simulink model "power_mosfet_device"  (R2025b)
settings: Solver=ode23tb  StartTime=0.0  StopTime=simlength  MaxStep=tc  RelTol=1e-3
values from neighbouring files (symbols this model uses):
  freq = 20e3    (= 20000)    [init_model.m]
  m = 0.5    [init_model.m]
  Rgate_turn_off = 1e-3    (= 0.001)    [init_model.m]
  Rgate_turn_on = 1    [init_model.m]
undefined symbols (not defined in the file or in its folder): cp_al, DThs_init, mosfet, Rth_mosfet_HA, Tambient, weigth
libraries: fl_lib x68, nesl_utility x32, simulink x4, advanced_mosfet_lib x2, basic_mosfet_lib x1, ee_lib x1
(part 2 of 2)

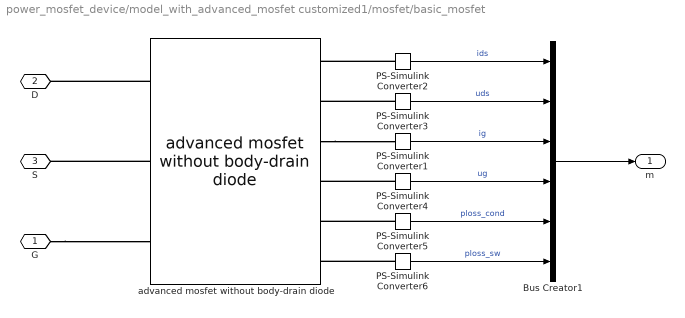
== system power_mosfet_device/model_with_advanced_mosfet customized1/mosfet/basic_mosfet ==
  Bus Creator1 : BusCreator  Inputs=6
  PS-Simulink Converter1 : nesl_utility/PS-Simulink Converter  PhysicalDomain=network_engine_domain  SubClassName=ps_output  LeftPortType=input  RightPortType=output  PseudoPeriodic=off  Frequencies=[]  VectorFormat=1-D array  Unit=A  AffineConversion=off
  PS-Simulink Converter2 : nesl_utility/PS-Simulink Converter  PhysicalDomain=network_engine_domain  SubClassName=ps_output  LeftPortType=input  RightPortType=output  PseudoPeriodic=off  Frequencies=[]  VectorFormat=1-D array  Unit=A  AffineConversion=off
  PS-Simulink Converter3 : nesl_utility/PS-Simulink Converter  PhysicalDomain=network_engine_domain  SubClassName=ps_output  LeftPortType=input  RightPortType=output  PseudoPeriodic=off  Frequencies=[]  VectorFormat=1-D array  Unit=V  AffineConversion=off
  PS-Simulink Converter4 : nesl_utility/PS-Simulink Converter  PhysicalDomain=network_engine_domain  SubClassName=ps_output  LeftPortType=input  RightPortType=output  PseudoPeriodic=off  Frequencies=[]  VectorFormat=1-D array  Unit=V  AffineConversion=off
  PS-Simulink Converter5 : nesl_utility/PS-Simulink Converter  PhysicalDomain=network_engine_domain  SubClassName=ps_output  LeftPortType=input  RightPortType=output  PseudoPeriodic=off  Frequencies=[]  VectorFormat=1-D array  Unit=W  AffineConversion=off
  PS-Simulink Converter6 : nesl_utility/PS-Simulink Converter  PhysicalDomain=network_engine_domain  SubClassName=ps_output  LeftPortType=input  RightPortType=output  PseudoPeriodic=off  Frequencies=[]  VectorFormat=1-D array  Unit=W  AffineConversion=off
  advanced mosfet without body-drain diode : advanced_mosfet_lib/advanced mosfet without body-drain diode  Vth=Vth_m V  g_fs=g_fs_m A/V  Rds_on=Rds_on_m Ohm  Cgs=Cgs_m F  Cgd=Cgd_m F  Cds=Cds_m F  Rg=Rgate_internal_m Ohm  Eon=Eon_m J  Eoff=Eoff_m J  Err=Err_m J  Voff_sw_loss=Voff_sw_loss_m V  Ion_sw_loss=Ion_sw_loss_m A  ids_i_specify=off  ids_i_priority=None  ids_i=0 A  ids_i_nominal_specify=off  ids_i_nominal_value=1  ids_i_nominal_unit=A  ids_ii_specify=off  ids_ii_priority=None  ids_ii=0 A  ids_ii_nominal_specify=off  ids_ii_nominal_value=1  ids_ii_nominal_unit=A  idsi_specify=off  idsi_priority=High  idsi=0 A  idsi_nominal_specify=off  idsi_nominal_value=1  idsi_nominal_unit=A  icgs_specify=off  icgs_priority=None  icgs=0 A  icgs_nominal_specify=off  icgs_nominal_value=1  icgs_nominal_unit=A  icgd_specify=off  icgd_priority=None  icgd=0 A  icgd_nominal_specify=off  icgd_nominal_value=1  icgd_nominal_unit=A  icds_specify=off  icds_priority=None  icds=0 A  icds_nominal_specify=off  icds_nominal_value=1  icds_nominal_unit=A  ugs_specify=off  ugs_priority=None  ugs=0 V  ugs_nominal_specify=off  ugs_nominal_value=1  ugs_nominal_unit=V  uds_specify=off  uds_priority=None  uds=0 V  uds_nominal_specify=off  uds_nominal_value=1  uds_nominal_unit=V  ucgs_specify=off  ucgs_priority=None  ucgs=0 V  ucgs_nominal_specify=off  ucgs_nominal_value=1  ucgs_nominal_unit=V  ucgd_specify=off  ucgd_priority=None  ucgd=0 V  ucgd_nominal_specify=off  ucgd_nominal_value=1  ucgd_nominal_unit=V  udsi_specify=off  udsi_priority=None  udsi=0 V  udsi_nominal_specify=off  udsi_nominal_value=1  udsi_nominal_unit=V  igs_specify=off  igs_priority=High  igs=0 A  igs_nominal_specify=off  igs_nominal_value=1  igs_nominal_unit=A  idsi_active_specify=off  idsi_active_priority=None  idsi_active=0 A  idsi_active_nominal_specify=off  idsi_active_nominal_value=1  idsi_active_nominal_unit=A  idsi_on_specify=off  idsi_on_priority=None  idsi_on=0 A  idsi_on_nominal_specify=off  idsi_on_nominal_value=1  idsi_on_nominal_unit=A
      settings: InternalSimscapePortConfiguration="{\"Bottom\":[],\"Left\":[{\"id\":\"D\",\"label\":\"D\",\"type\":\"foundation.electrical.electrical\"},{\"id\":\"S\",\"label\":\"S\",\"type\":\"foundation.electrical.electrical\"},{\"id\":\"G\",\"label\":\"G\",\"type\":\"foundation.electrical.electrical\"}],\"Right\":[{\"id\":\"idsi_out\",\"label\":\"ids\",\"type\":\"output\"},{\"id\":\"udsi_out\",\"label\":\"uds\",\"type\":\"output\"},{\"id\":\"igs_out\",\"label\":\"igs\",\"type\":\"output\"},{\"id\":\"ugs_out\",\"label\":\"ugs\",\"type\":\"output\"},{\"id\":\"ploss_cond\",\"label\":\"ploss_cond\",\"type\":\"output\"},{\"id\":\"ploss_sw\",\"label\":\"ploss_sw\",\"type\":\"output\"}],\"Top\":[]}"
  G : PMIOPort  Side=Left
  D : PMIOPort  Port=2  Side=Left
  S : PMIOPort  Port=3  Side=Right
  m : Outport
  wires:
  PS-Simulink Converter6/1 -> Bus Creator1/6  "ploss_sw"
  PS-Simulink Converter5/1 -> Bus Creator1/5  "ploss_cond"
  PS-Simulink Converter4/1 -> Bus Creator1/4  "ug"
  PS-Simulink Converter1/1 -> Bus Creator1/3  "ig"
  PS-Simulink Converter3/1 -> Bus Creator1/2  "uds"
  PS-Simulink Converter2/1 -> Bus Creator1/1  "ids"
  Bus Creator1/1 -> m/1
  connections:
  PS-Simulink Converter6/LConn1 -- advanced mosfet without body-drain diode/RConn6
  PS-Simulink Converter5/LConn1 -- advanced mosfet without body-drain diode/RConn5
  advanced mosfet without body-drain diode/RConn3 -- PS-Simulink Converter1/LConn1
  PS-Simulink Converter4/LConn1 -- advanced mosfet without body-drain diode/RConn4
  G/RConn1 -- advanced mosfet without body-drain diode/LConn3
  advanced mosfet without body-drain diode/LConn2 -- S/RConn1
  advanced mosfet without body-drain diode/LConn1 -- D/RConn1
  PS-Simulink Converter2/LConn1 -- advanced mosfet without body-drain diode/RConn1
  PS-Simulink Converter3/LConn1 -- advanced mosfet without body-drain diode/RConn2

== system power_mosfet_device/model_with_basic_mosfet/mosfet/basic_mosfet ==
  Bus Creator1 : BusCreator  Inputs=2
  PS-Simulink Converter2 : nesl_utility/PS-Simulink Converter  PhysicalDomain=network_engine_domain  SubClassName=ps_output  LeftPortType=input  RightPortType=output  PseudoPeriodic=off  Frequencies=[]  VectorFormat=1-D array  Unit=A  AffineConversion=off
  PS-Simulink Converter3 : nesl_utility/PS-Simulink Converter  PhysicalDomain=network_engine_domain  SubClassName=ps_output  LeftPortType=input  RightPortType=output  PseudoPeriodic=off  Frequencies=[]  VectorFormat=1-D array  Unit=V  AffineConversion=off
  basic mosfet : basic_mosfet_lib/basic mosfet  Vth=Vth V  g_fs=g_fs A/V  Rds_on=Rds_on Ohm  ids_specify=off  ids_priority=High  ids=0 A  ids_nominal_specify=off  ids_nominal_value=1  ids_nominal_unit=A  uds_specify=off  uds_priority=None  uds=0 V  uds_nominal_specify=off  uds_nominal_value=1  uds_nominal_unit=V  ib_specify=off  ib_priority=None  ib=0 A  ib_nominal_specify=off  ib_nominal_value=1  ib_nominal_unit=A  ids_on_specify=off  ids_on_priority=None  ids_on=0 A  ids_on_nominal_specify=off  ids_on_nominal_value=1  ids_on_nominal_unit=A
      settings: InternalSimscapePortConfiguration="{\"Bottom\":[],\"Left\":[{\"id\":\"D\",\"label\":\"D\",\"type\":\"foundation.electrical.electrical\"},{\"id\":\"S\",\"label\":\"S\",\"type\":\"foundation.electrical.electrical\"},{\"id\":\"ugs\",\"label\":\"ugs\",\"type\":\"input\"}],\"Right\":[{\"id\":\"ids_out\",\"label\":\"ids\",\"type\":\"output\"},{\"id\":\"uds_out\",\"label\":\"uds\",\"type\":\"output\"}],\"Top\":[]}"
  ugs : PMIOPort  Side=Left
  D : PMIOPort  Port=2  Side=Left
  S : PMIOPort  Port=3  Side=Right
  m : Outport
  wires:
  PS-Simulink Converter3/1 -> Bus Creator1/2  "uds"
  PS-Simulink Converter2/1 -> Bus Creator1/1  "ids"
  Bus Creator1/1 -> m/1
  connections:
  basic mosfet/LConn3 -- ugs/RConn1
  basic mosfet/LConn1 -- D/RConn1
  PS-Simulink Converter2/LConn1 -- basic mosfet/RConn1
  basic mosfet/LConn2 -- S/RConn1
  PS-Simulink Converter3/LConn1 -- basic mosfet/RConn2

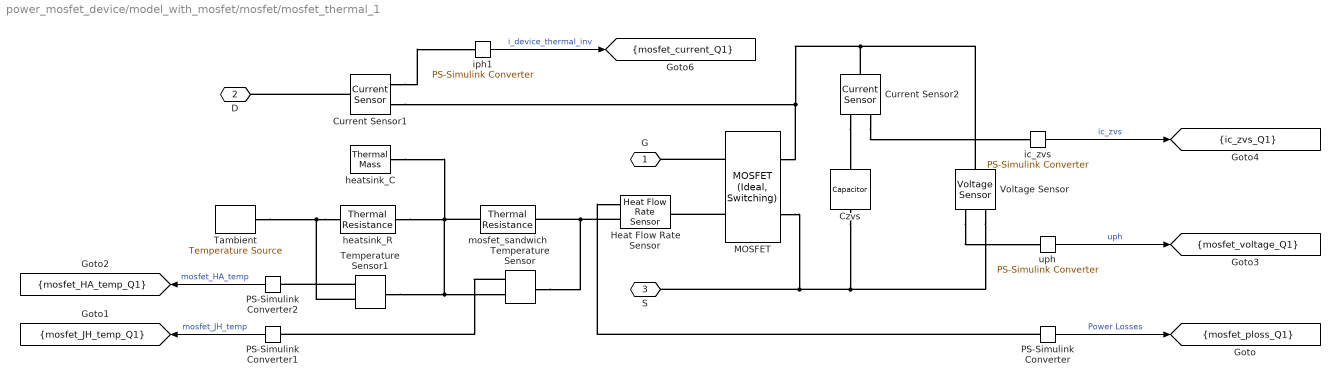
== system power_mosfet_device/model_with_mosfet/mosfet/mosfet_thermal_1 ==
  Current Sensor1 : fl_lib/Electrical/Electrical Sensors/Current Sensor
  Current Sensor2 : fl_lib/Electrical/Electrical Sensors/Current Sensor
  Czvs : fl_lib/Electrical/Electrical Elements/Capacitor  c=Csnubber F  r=Rsnubber Ohm  g=0 1/Ohm  i_specify=off  i_priority=None  i=0 A  i_nominal_specify=off  i_nominal_value=1  i_nominal_unit=A  v_specify=off  v_priority=None  v=0 V  v_nominal_specify=off  v_nominal_value=1  v_nominal_unit=V  vc_specify=off  vc_priority=High  vc=0 V  vc_nominal_specify=off  vc_nominal_value=1  vc_nominal_unit=V
  Heat Flow Rate Sensor : fl_lib/Thermal/Thermal Sensors/Heat Flow Rate Sensor
  MOSFET : ee_lib/Semiconductors & Converters/MOSFET (Ideal, Switching)  port_option=ee.enum.controlport.ps  Rds=Rds_on Ohm  Goff=1e-6 1/Ohm  Vth=Vth V  diode_param=ee.enum.converters.protectiondiode.nodynamics  diode_Vf=Vdon_diode V  diode_Ron=Rdon_diode Ohm  diode_Goff=1e-5 1/Ohm  diode_C=50e-9 F  diode_iRM=-235 A  diode_iF=300 A  diode_idot=-50 A/us  diode_trr_param=ee.enum.converters.diodeReverseParam.trr_factor  diode_trr_factor=3  diode_trr=15 us  diode_Qrr=1500 s*uA  ids_specify=off  ids_priority=None  ids=0 A  ids_nominal_specify=off  ids_nominal_value=1  ids_nominal_unit=A  vds_specify=off  vds_priority=None  vds=0 V  vds_nominal_specify=off  vds_nominal_value=1  vds_nominal_unit=V  vgs_specify=off  vgs_priority=None  vgs=0 V  vgs_nominal_specify=off  vgs_nominal_value=1  vgs_nominal_unit=V  thermal_loss_option=ee.enum.converters.thermalLossOption.constantvalues  Von_data=[0, 1.8, 3.2, 6, 10, 16; 0, 2, 5.5, 9.5, 15, 25] V  Tj=[298.15, 448.15] K  Iout_data=[0, 20, 40, 60, 80, 100] A  Eon_data=[0, 55.04, 124.57, 235.53, 362.12; 0, 71.25, 161.25, 304.88, 468.75] * 1e-6 J  Eoff_data=[0, 18, 30, 56.1, 76.5; 0, 22.5, 37.5, 70.13, 95.63] * 1e-6 J  Eon_data_3D=[zeros(2, 5, 3)] J  Eoff_data_3D=[zeros(2, 5, 3)] J  Tj_loss=[298.15, 448.15] K  Iout_data_loss=[0, 10, 20, 30, 40] A  tabulateWithVds=false  Vds_loss=[0, 150, 300] V  Eon_scalar=Eon J  Eoff_scalar=Eoff J  Voff=Voff_sw_loss V  Iout_scalar=Ion_sw_loss A  useCurrentFromPreviousCycle=true  useVoltageFromPreviousCycle=true  diodeModelType=ee.enum.converters.diodeModelType.pwl  diodeTableType=ee.enum.diode.tableType.IfMat  diode_ReverseIVType=ee.enum.diode.diodeReverseIV.constant  diode_IfMat=[.07, .12, .19, 1.75, 4.24, 7.32, 11.2; .16, .3, .72, 2.14, 4.02, 6.35, 9.12] A  diode_VfMat=[.9, 1.15, 1.25, 1.5, 1.75, 2.17, 2.6, 2.85; .58, .68, .75, 1.1, 1.38, 1.77, 2.27, 2.7] V  diode_TjVec=[25, 125] degC  diode_VfVec=[.5, .7, .9, 1.3, 1.7, 2.1, 2.5] V  diode_IfVec=[.1, .2, .5, 1, 2, 4, 7, 10] A  diode_IrMat=[1e-06, 2e-06, 5e-06, 1e-05, 2.5e-05, 5e-05, .0001; 2e-06, 5e-06, 1e-05, 4e-05, 8e-05, .0002, .0005] A  diode_VrMat=[10, 100, 200, 250, 300, 325, 350; 10, 70, 160, 220, 270, 300, 320] V  diode_VrVec=[10, 20, 40, 50, 70, 80, 100] V  diode_IrVec=[1e-06, 2e-06, 5e-06, 1e-05, 2e-05, 5e-05, .0001] A  diode_Vr=-600 V  diode_Ls=150 nH  diode_Erec=0.03 J  diode_rec_loss_model=ee.enum.diode.reverseRecoveryModel.fixed  diode_ErecVal=0 J  diode_scaleWithIandV=false  diode_ErecMat=zeros(2, 3) J  diode_TjrecVec=[298.15, 398.15] K  diode_IfrecVec=[.1, 1, 10] A  diode_IrecVal=10 A  diode_VrecVal=10 V  diode_tFilter=1 / 1000 / 100 s  separateThermalPortForDiode=false  thermal_network_parameterization=ee.enum.thermalNetworkTopology.external  Rth=[.03, .2] K/W  Rth_Cauer=[.03, .1, .2] K/W  Rth_Foster=[.03, .2] K/W  thermal_mass_parameterization=ee.enum.thermalNetwork.thermalmass  thermal_mass=[3, 25] J/K  thermal_mass_Cauer=[3, 10, 25] J/K  thermal_mass_Foster=[33, 50] J/K  thermal_time_constant=[.1, 5] s  thermal_time_constant_Cauer=[.1, 1, 5] s  thermal_time_constant_Foster=[1, 10] s  thermal_mass_initial_temperatures=[80, 80] degC  thermal_mass_initial_temperatures_Cauer=[25, 25, 25] degC  junction_thermal_mass=JunctionTermalMass J/K  Tvec_initial_Foster=[25, 25, 25, 25] degC  RthDiode=[.03, .2] K/W  RthCauerDiode=[.03, .1, .2] K/W  RthFosterDiode=[.03, .2] K/W  thermalMassDiode=[3, 25] J/K  thermalMassCauerDiode=[3, 10, 25] J/K  thermalMassFosterDiode=[33, 50] J/K  thermalTauDiode=[.1, 5] s  thermalTauCauerDiode=[.1, 1, 5] s  thermalTauFosterDiode=[1, 10] s  thermalMassInitTempDiode=[25, 25] degC  thermalMassInitTempCauerDiode=[25, 25, 25] degC  junctionthermalMassDiode=0.1 J/K  TVecInitialFosterDiode=[25, 25, 25, 25] degC  no_thermal_network=0  mosfet_junction_temperature_specify=on  mosfet_junction_temperature_priority=High  mosfet_junction_temperature=Tambient+DThs_init degC  mosfet_junction_temperature_nominal_specify=off  mosfet_junction_temperature_nominal_value=1  mosfet_junction_temperature_nominal_unit=degC  diode_junction_temperature_specify=off  diode_junction_temperature_priority=None  diode_junction_temperature=25 degC  diode_junction_temperature_nominal_specify=off  diode_junction_temperature_nominal_value=1  diode_junction_temperature_nominal_unit=degC  Qj_specify=off  Qj_priority=None  Qj=0 W  Qj_nominal_specify=off  Qj_nominal_value=1  Qj_nominal_unit=W  accumulatedSwitchingLosses_specify=off  accumulatedSwitchingLosses_priority=None  accumulatedSwitchingLosses=0 J
      settings: InternalSimscapePortConfiguration="{\"Bottom\":[],\"Left\":[{\"id\":\"G\",\"label\":\"\",\"type\":\"input\"},{\"id\":\"H\",\"label\":\"\",\"type\":\"foundation.thermal.thermal\"}],\"Right\":[{\"id\":\"D\",\"label\":\"\",\"type\":\"foundation.electrical.electrical\"},{\"id\":\"S\",\"label\":\"\",\"type\":\"foundation.electrical.electrical\"}],\"Top\":[]}"
  PS-Simulink Converter : nesl_utility/PS-Simulink Converter  PhysicalDomain=network_engine_domain  SubClassName=ps_output  LeftPortType=input  RightPortType=output  PseudoPeriodic=off  Frequencies=[]  VectorFormat=1-D array  Unit=W  AffineConversion=off
  PS-Simulink Converter1 : nesl_utility/PS-Simulink Converter  PhysicalDomain=network_engine_domain  SubClassName=ps_output  LeftPortType=input  RightPortType=output  PseudoPeriodic=off  Frequencies=[]  VectorFormat=1-D array  Unit=degC  AffineConversion=off
  PS-Simulink Converter2 : nesl_utility/PS-Simulink Converter  PhysicalDomain=network_engine_domain  SubClassName=ps_output  LeftPortType=input  RightPortType=output  PseudoPeriodic=off  Frequencies=[]  VectorFormat=1-D array  Unit=degC  AffineConversion=off
  Tambient : fl_lib/Thermal/Thermal Sources/Temperature Source  temperature=Tambient degC
  Temperature Sensor : fl_lib/Thermal/Thermal Sensors/Temperature Sensor  temperature_measure=foundation.enum.MeasurementReference.difference
  Temperature Sensor1 : fl_lib/Thermal/Thermal Sensors/Temperature Sensor  temperature_measure=foundation.enum.MeasurementReference.difference
  Voltage Sensor : fl_lib/Electrical/Electrical Sensors/Voltage Sensor
  heatsink_C : fl_lib/Thermal/Thermal Elements/Thermal Mass  mass_type=foundation.enum.constant_variable.constant  mass=mass_heatsink kg  sp_heat=specific_heat J/(K*kg)  mass_min=1e-6 kg  num_ports=foundation.enum.numPorts2.one  m_specify=off  m_priority=High  m=1 kg  m_nominal_specify=off  m_nominal_value=1  m_nominal_unit=kg  T_specify=on  T_priority=High  T=DThs_init+Tambient degC  T_nominal_specify=off  T_nominal_value=1  T_nominal_unit=K  Q_specify=off  Q_priority=High  Q=0 W  Q_nominal_specify=off  Q_nominal_value=1  Q_nominal_unit=W
  heatsink_R : fl_lib/Thermal/Thermal Elements/Thermal Resistance  resistance=rth_mosfet_HA K/W  T_specify=off  T_priority=High  T=0 deltadegC  T_nominal_specify=off  T_nominal_value=1  T_nominal_unit=K  Q_specify=off  Q_priority=None  Q=0 W  Q_nominal_specify=off  Q_nominal_value=1  Q_nominal_unit=W
  ic_zvs : nesl_utility/PS-Simulink Converter  PhysicalDomain=network_engine_domain  SubClassName=ps_output  LeftPortType=input  RightPortType=output  PseudoPeriodic=off  Frequencies=[]  VectorFormat=1-D array  Unit=A  AffineConversion=off
  iph1 : nesl_utility/PS-Simulink Converter  PhysicalDomain=network_engine_domain  SubClassName=ps_output  LeftPortType=input  RightPortType=output  PseudoPeriodic=off  Frequencies=[]  VectorFormat=1-D array  Unit=A  AffineConversion=off
  mosfet_sandwich : fl_lib/Thermal/Thermal Elements/Thermal Resistance  resistance=rth_mosfet_JH K/W  T_specify=off  T_priority=High  T=0 degC  T_nominal_specify=off  T_nominal_value=1  T_nominal_unit=K  Q_specify=off  Q_priority=None  Q=0 W  Q_nominal_specify=off  Q_nominal_value=1  Q_nominal_unit=W
  uph : nesl_utility/PS-Simulink Converter  PhysicalDomain=network_engine_domain  SubClassName=ps_output  LeftPortType=input  RightPortType=output  PseudoPeriodic=off  Frequencies=[]  VectorFormat=1-D array  Unit=V  AffineConversion=off
  G : PMIOPort  Side=Left
  D : PMIOPort  Port=2  Side=Left
  S : PMIOPort  Port=3  Side=Right
  tag scope: ic_zvs_Q1=scoped, mosfet_HA_temp_Q1=scoped, mosfet_JH_temp_Q1=scoped, mosfet_current_Q1=scoped, mosfet_ploss_Q1=scoped, mosfet_voltage_Q1=scoped
  wires:
  ic_zvs/1 -> [ic_zvs_Q1]  "ic_zvs"
  uph/1 -> [mosfet_voltage_Q1]  "uph"
  iph1/1 -> [mosfet_current_Q1]  "i_device_thermal_inv"
  PS-Simulink Converter1/1 -> [mosfet_JH_temp_Q1]  "mosfet_JH_temp"
  PS-Simulink Converter2/1 -> [mosfet_HA_temp_Q1]  "mosfet_HA_temp"
  PS-Simulink Converter/1 -> [mosfet_ploss_Q1]  "Power Losses"
  connections:
  Current Sensor2/RConn1 -- ic_zvs/LConn1
  Current Sensor2/RConn2 -- Czvs/LConn1
  Voltage Sensor/RConn1 -- uph/LConn1
  Current Sensor1/RConn1 -- iph1/LConn1
  MOSFET/RConn1 -- Voltage Sensor/LConn1 -- Current Sensor2/LConn1 -- Current Sensor1/RConn2
  Current Sensor1/LConn1 -- D/RConn1
  MOSFET/LConn2 -- Heat Flow Rate Sensor/LConn1
  Temperature Sensor1/RConn2 -- PS-Simulink Converter2/LConn1
  heatsink_R/RConn1 -- Temperature Sensor1/RConn1 -- Tambient/LConn1
  Temperature Sensor/RConn2 -- PS-Simulink Converter1/LConn1
  heatsink_C/LConn1 -- heatsink_R/LConn1 -- Temperature Sensor/RConn1 -- Temperature Sensor1/LConn1 -- mosfet_sandwich/RConn1
  mosfet_sandwich/LConn1 -- Heat Flow Rate Sensor/RConn2 -- Temperature Sensor/LConn1
  PS-Simulink Converter/LConn1 -- Heat Flow Rate Sensor/RConn1
  MOSFET/LConn1 -- G/RConn1
  MOSFET/RConn2 -- Voltage Sensor/RConn2 -- Czvs/RConn1 -- S/RConn1
